simulink model "Comau_endeff_Comp"  (R2024b)
settings: Solver=FixedStepAuto  StartTime=0.0  StopTime=inf  FixedStep=Ts  RelTol=1e-3
model workspace (MATLAB code in the model file):
  | %% SMART_5NJ_110_3_0_DataFile
  | %============= RigidTransform =============%
  | 
  | %Initialize the RigidTransform structure array by filling in null values.
  | smiDataRobot.RigidTransform(16).translation = [0.0 0.0 0.0];
  | smiDataRobot.RigidTransform(16).angle = 0.0;
  | smiDataRobot.RigidTransform(16).axis = [0.0 0.0 0.0];
  | smiDataRobot.RigidTransform(16).ID = "";
  | 
  | %Translation Method - Cartesian
  | %Rotation Method - Arbitrary Axis
  | smiDataRobot.RigidTransform(1).translation = [0 331 0];  % mm
  | smiDataRobot.RigidTransform(1).angle = 0;  % rad
  | smiDataRobot.RigidTransform(1).axis = [0 0 0];
  | smiDataRobot.RigidTransform(1).ID = "AssemblyGround[SMART-5 NJ-110-3.0 (3D-STEP).STEP-1:SMART-5 NJ-110-3.0_p02.STEP-1]";
  | 
  | %Translation Method - Cartesian
  | %Rotation Method - Arbitrary Axis
  | smiDataRobot.RigidTransform(2).translation = [-450 2240 0];  % mm
  | smiDataRobot.RigidTransform(2).angle = 0;  % rad
  | smiDataRobot.RigidTransform(2).axis = [0 0 0];
  | smiDataRobot.RigidTransform(2).ID = "AssemblyGround[SMART-5 NJ-110-3.0 (3D-STEP).STEP-1:SMART-5 NJ-110-3.0_p05.STEP-1]";
  | 
  | %Translation Method - Cartesian
  | %Rotation Method - Arbitrary Axis
  | smiDataRobot.RigidTransform(3).translation = [-350 830 294.75];  % mm
  | smiDataRobot.RigidTransform(3).angle = 3.1415926535897931;  % rad
  | smiDataRobot.RigidTransform(3).axis = [1 0 0];
  | smiDataRobot.RigidTransform(3).ID = "AssemblyGround[SMART-5 NJ-110-3.0 (3D-STEP).STEP-1:SMART-5 NJ-110-3.0_CR82350080_SM.STEP-1]";
  | 
  | %Translation Method - Cartesian
  | %Rotation Method - Arbitrary Axis
  | smiDataRobot.RigidTransform(4).translation = [-1842.1799999999998 2240 9.9999999999999998e-13];  % mm
  | smiDataRobot.RigidTransform(4).angle = 0;  % rad
  | smiDataRobot.RigidTransform(4).axis = [0 0 0];
  | smiDataRobot.RigidTransform(4).ID = "AssemblyGround[SMART-5 NJ-110-3.0 (3D-STEP).STEP-1:SMART-5 NJ-110-3.0_p08.STEP-1]";
  | 
  | %Translation Method - Cartesian
  | %Rotation Method - Arbitrary Axis
  | smiDataRobot.RigidTransform(5).translation = [-1917.4300000000001 2240 -4.9999999999999997e-12];  % mm
  | smiDataRobot.RigidTransform(5).angle = 1.5707963267948977;  % rad
  | smiDataRobot.RigidTransform(5).axis = [-1.4999999999999981e-15 -1 -1.4999999999999981e-15];
  | smiDataRobot.RigidTransform(5).ID = "AssemblyGround[SMART-5 NJ-110-3.0 (3D-STEP).STEP-1:SMART-5 NJ-110-3.0_CR82350030_SM.STEP-1]";
  | 
  | %Translation Method - Cartesian
  | %Rotation Method - Arbitrary Axis
  | smiDataRobot.RigidTransform(6).translation = [0 0 0];  % mm
  | smiDataRobot.RigidTransform(6).angle = 0;  % rad
  | smiDataRobot.RigidTransform(6).axis = [0 0 0];
  | smiDataRobot.RigidTransform(6).ID = "AssemblyGround[SMART-5 NJ-110-3.0 (3D-STEP).STEP-1:SMART-5 NJ-110-3.0_p01.STEP-1]";
  | 
  | %Translation Method - Cartesian
  | %Rotation Method - Arbitrary Axis
  | smiDataRobot.RigidTransform(7).translation = [-240.25 2190 169.72568626429799];  % mm
  | smiDataRobot.RigidTransform(7).angle = 2.0943951023931966;  % rad
  | smiDataRobot.RigidTransform(7).axis = [0.57735026918962562 -0.57735026918962606 -0.57735026918962562];
  | smiDataRobot.RigidTransform(7).ID = "AssemblyGround[SMART-5 NJ-110-3.0 (3D-STEP).STEP-1:SMART-5 NJ-110-3.0_CR82350050_SM.STEP-1]";
  | 
  | %Translation Method - Cartesian
  | %Rotation Method - Arbitrary Axis
  | smiDataRobot.RigidTransform(8).translation = [-350 830 135.5];  % mm
  | smiDataRobot.RigidTransform(8).angle = 0;  % rad
  | smiDataRobot.RigidTransform(8).axis = [0 0 0];
  | smiDataRobot.RigidTransform(8).ID = "AssemblyGround[SMART-5 NJ-110-3.0 (3D-STEP).STEP-1:SMART-5 NJ-110-3.0_p03.STEP-1]";
  | 
  | %Translation Method - Cartesian
  | %Rotation Method - Arbitrary Axis
  | smiDataRobot.RigidTransform(9).translation = [-350 830 -350.25];  % mm
  | smiDataRobot.RigidTransform(9).angle = 3.1415926535897913;  % rad
  | smiDataRobot.RigidTransform(9).axis = [-0 -0 -1];
  | smiDataRobot.RigidTransform(9).ID = "AssemblyGround[SMART-5 NJ-110-3.0 (3D-STEP).STEP-1:SMART-5 NJ-110-3.0_CR82350070_SM.STEP-2]";
  | 
  | %Translation Method - Cartesian
  | %Rotation Method - Arbitrary Axis
  | smiDataRobot.RigidTransform(10).translation = [-31.217696610640999 802.11016232075008 -179.5];  % mm
  | smiDataRobot.RigidTransform(10).angle = 0;  % rad
  | smiDataRobot.RigidTransform(10).axis = [0 0 0];
  | smiDataRobot.RigidTransform(10).ID = "AssemblyGround[SMART-5 NJ-110-3.0 (3D-STEP).STEP-1:SMART-5 NJ-110-3.0_p06.STEP-1]";
  | 
  | %Translation Method - Cartesian
  | %Rotation Method - Arbitrary Axis
  | smiDataRobot.RigidTransform(11).translation = [-350 830 -194.5];  % mm
  | smiDataRobot.RigidTransform(11).angle = 0.087266462599717279;  % rad
  | smiDataRobot.RigidTransform(11).axis = [0 -1.1451882774215491e-14 -1];
  | smiDataRobot.RigidTransform(11).ID = "AssemblyGround[SMART-5 NJ-110-3.0 (3D-STEP).STEP-1:SMART-5 NJ-110-3.0_p04.STEP-1]";
  | 
  | %Translation Method - Cartesian
  | %Rotation Method - Arbitrary Axis
  | smiDataRobot.RigidTransform(12).translation = [-2007.179999999981 2240.0000000000132 -6.4999999999999995e-11];  % mm
  | smiDataRobot.RigidTransform(12).angle = 0;  % rad
  | smiDataRobot.RigidTransform(12).axis = [0 0 0];
  | smiDataRobot.RigidTransform(12).ID = "AssemblyGround[SMART-5 NJ-110-3.0 (3D-STEP).STEP-1:SMART-5 NJ-110-3.0_p10.STEP-1]";
  | 
  | %Translation Method - Cartesian
  | %Rotation Method - Arbitrary Axis
  | smiDataRobot.RigidTransform(13).translation = [156.75059808498401 472.5 90.5];  % mm
  | smiDataRobot.RigidTransform(13).angle = 2.7734925708571119;  % rad
  | smiDataRobot.RigidTransform(13).axis = [0.1861567878973851 0.69474659060686583 -0.69474659060686583];
  | smiDataRobot.RigidTransform(13).ID = "AssemblyGround[SMART-5 NJ-110-3.0 (3D-STEP).STEP-1:SMART-5 NJ-110-3.0_CR82350070_SM.STEP-1]";
  | 
  | %Translation Method - Cartesian
  | %Rotation Method - Arbitrary Axis
  | smiDataRobot.RigidTransform(14).translation = [-1967.1799999999998 2239.9999999999964 -2.5000000000000001e-11];  % mm
  | smiDataRobot.RigidTransform(14).angle = 1.5707963267948954;  % rad
  | smiDataRobot.RigidTransform(14).axis = [-4.5000000000000005e-15 1 3.5000000000000001e-15];
  | smiDataRobot.RigidTransform(14).ID = "AssemblyGround[SMART-5 NJ-110-3.0 (3D-STEP).STEP-1:SMART-5 NJ-110-3.0_p09.STEP-1]";
  | 
  | %Translation Method - Cartesian
  | %Rotation Method - Arbitrary Axis
  | smiDataRobot.RigidTransform(15).translation = [-495 2239.9999999999982 -2.5000000000000001e-11];  % mm
  | smiDataRobot.RigidTransform(15).angle = 2.0943951023932024;  % rad
  | smiDataRobot.RigidTransform(15).axis = [-0.57735026918962851 -0.57735026918962118 0.57735026918962751];
  | smiDataRobot.RigidTransform(15).ID = "AssemblyGround[SMART-5 NJ-110-3.0 (3D-STEP).STEP-1:SMART-5 NJ-110-3.0_p07.STEP-1]";
  | 
  | %Translation Method - Cartesian
  | %Rotation Method - Arbitrary Axis
  | smiDataRobot.RigidTransform(16).translation = [0 0 0];  % mm
  | smiDataRobot.RigidTransform(16).angle = 0;  % rad
  | smiDataRobot.RigidTransform(16).axis = [0 0 0];
  | smiDataRobot.RigidTransform(16).ID = "RootGround[SMART-5 NJ-110-3.0 (3D-STEP).STEP-1]";
  | 
  | 
  | %============= Solid =============%
  | %Center of Mass (CoM) %Moments of Inertia (MoI) %Product of Inertia (PoI)
  | 
  | %Initialize the Solid structure array by filling in null values.
  | smiDataRobot.Solid(14).mass = 0.0;
  | smiDataRobot.Solid(14).CoM = [0.0 0.0 0.0];
  | smiDataRobot.Solid(14).MoI = [0.0 0.0 0.0];
  | smiDataRobot.Solid(14).PoI = [0.0 0.0 0.0];
  | smiDataRobot.Solid(14).color = [0.0 0.0 0.0];
  | smiDataRobot.Solid(14).opacity = 0.0;
  | smiDataRobot.Solid(14).ID = "";
  | 
  | %Inertia Type - Custom
  | %Visual Properties - Simple
  | smiDataRobot.Solid(1).mass = 52.706031176315982;  % kg
  | smiDataRobot.Solid(1).CoM = [-242.66897813542667 296.14549865714821 12.560965025190244];  % mm
  | smiDataRobot.Solid(1).MoI = [4136639.3686790983 3647453.6565928138 4173251.5664203875];  % kg*mm^2
  | smiDataRobot.Solid(1).PoI = [21269.015167562859 -54887.133975236575 1321088.2058438642];  % kg*mm^2
  | smiDataRobot.Solid(1).color = [0.203 0.210 0.239];
  | smiDataRobot.Solid(1).opacity = 1;
  | smiDataRobot.Solid(1).ID = "SMART-5 NJ-110-3.0_p02.STEP*:*Default";
  | 
  | %Inertia Type - Custom
  | %Visual Properties - Simple
  | smiDataRobot.Solid(2).mass = 25.314195721014904;  % kg
  | smiDataRobot.Solid(2).CoM = [81.922886858874577 -33.833989402443976 14.448782406787638];  % mm
  | smiDataRobot.Solid(2).MoI = [783008.26269064494 548584.67016851983 525604.1322728931];  % kg*mm^2
  | smiDataRobot.Solid(2).PoI = [-112599.38170428496 21299.174138007162 72588.874515329284];  % kg*mm^2
  | smiDataRobot.Solid(2).color = [0.792156862745098 0.81960784313725488 0.93333333333333335];
  | smiDataRobot.Solid(2).opacity = 1;
  | smiDataRobot.Solid(2).ID = "SMART-5 NJ-110-3.0_p05.STEP*:*Default";
  | 
  | %Inertia Type - Custom
  | %Visual Properties - Simple
  | smiDataRobot.Solid(3).mass = 9.4493198216073964;  % kg
  | smiDataRobot.Solid(3).CoM = [0.00035605587580101627 0.59254727846081734 -131.34248514352112];  % mm
  | smiDataRobot.Solid(3).MoI = [96683.905101085853 96090.527287838268 47612.014811029614];  % kg*mm^2
  | smiDataRobot.Solid(3).PoI = [678.15178926669853 -1.9373731491872181 -0.37884372181229253];  % kg*mm^2
  | smiDataRobot.Solid(3).color = [0.792156862745098 0.81960784313725488 0.93333333333333335];
  | smiDataRobot.Solid(3).opacity = 1;
  | smiDataRobot.Solid(3).ID = "SMART-5 NJ-110-3.0_CR82350080_SM.STEP*:*Default";
  | 
  | %Inertia Type - Custom
  | %Visual Properties - Simple
  | smiDataRobot.Solid(4).mass = 27.907822986627043;  % kg
  | smiDataRobot.Solid(4).CoM = [176.91381036358237 3.8341896469272663 1.9754510358205102];  % mm
  | smiDataRobot.Solid(4).MoI = [482005.2410957645 820993.89522460627 552912.66986302414];  % kg*mm^2
  | smiDataRobot.Solid(4).PoI = [-5805.283149630598 -66627.605911827952 -6375.7492384737961];  % kg*mm^2
  | smiDataRobot.Solid(4).color = [0.792156862745098 0.81960784313725488 0.93333333333333335];
  | smiDataRobot.Solid(4).opacity = 1;
  | smiDataRobot.Solid(4).ID = "SMART-5 NJ-110-3.0_p08.STEP*:*Default";
  | 
  | %Inertia Type - Custom
  | %Visual Properties - Simple
  | smiDataRobot.Solid(5).mass = 1.8204370609575367;  % kg
  | smiDataRobot.Solid(5).CoM = [0.0011781120658499607 1.8532136422554566 -83.079832406507592];  % mm
  | smiDataRobot.Solid(5).MoI = [7475.3672830480818 7269.0527134527229 2858.8228291073215];  % kg*mm^2
  | smiDataRobot.Solid(5).PoI = [189.23833790092377 0.076539858692730889 -0.14274057644209939];  % kg*mm^2
  | smiDataRobot.Solid(5).color = [0.792156862745098 0.81960784313725488 0.93333333333333335];
  | smiDataRobot.Solid(5).opacity = 1;
  | smiDataRobot.Solid(5).ID = "SMART-5 NJ-110-3.0_CR82350030_SM.STEP*:*Default";
  | 
  | %Inertia Type - Custom
  | %Visual Properties - Simple
  | smiDataRobot.Solid(6).mass = 98.712536679746705;  % kg
  | smiDataRobot.Solid(6).CoM = [36.183943831325131 132.25114554111747 -0.030525648643372944];  % mm
  | smiDataRobot.Solid(6).MoI = [3268478.8711421788 6102276.4254572866 4269111.0143532446];  % kg*mm^2
  | smiDataRobot.Solid(6).PoI = [-35.583053939592197 631.47068636807955 -2524.4017230519235];  % kg*mm^2
  | smiDataRobot.Solid(6).color = [0.792156862745098 0.81960784313725488 0.93333333333333335];
  | smiDataRobot.Solid(6).opacity = 1;
  | smiDataRobot.Solid(6).ID = "SMART-5 NJ-110-3.0_p01.STEP*:*Default";
  | 
  | %Inertia Type - Custom
  | %Visual Properties - Simple
  | smiDataRobot.Solid(7).mass = 3.5666359355844257;  % kg
  | smiDataRobot.Solid(7).CoM = [1.2461000205248818 -0.0010192432622059655 -85.200466358919499];  % mm
  | smiDataRobot.Solid(7).MoI = [17145.157040564802 17509.336534066519 10295.619245635809];  % kg*mm^2
  | smiDataRobot.Solid(7).PoI = [-0.163954126982988 300.11359564551077 0.32104894325969818];  % kg*mm^2
  | smiDataRobot.Solid(7).color = [0.6392157 0.0 0.0];
  | smiDataRobot.Solid(7).opacity = 1;
  | smiDataRobot.Solid(7).ID = "SMART-5 NJ-110-3.0_CR82350050_SM.STEP*:*Default";
  | 
  | %Inertia Type - Custom
  | %Visual Properties - Simple
  | smiDataRobot.Solid(8).mass = 22.854890403146104;  % kg
  | smiDataRobot.Solid(8).CoM = [-23.928506665749911 523.99566525340538 -159.70044895169784];  % mm
  | smiDataRobot.Solid(8).MoI = [3177590.9155515293 341455.30737882649 3069690.399421786];  % kg*mm^2
  | smiDataRobot.Solid(8).PoI = [51188.540610659591 -6971.0396180961588 7197.3923801430437];  % kg*mm^2
  | smiDataRobot.Solid(8).color = [0.64 0.0 0.0];
  | smiDataRobot.Solid(8).opacity = 1;
  | smiDataRobot.Solid(8).ID = "SMART-5 NJ-110-3.0_p03.STEP*:*Default";
  | 
  | %Inertia Type - Custom
  | %Visual Properties - Simple
  | smiDataRobot.Solid(9).mass = 8.5814594224327365;  % kg
  | smiDataRobot.Solid(9).CoM = [0.00039190881468678792 0.65247306493897117 -117.33220651590989];  % mm
  | smiDataRobot.Solid(9).MoI = [76220.255867257161 75627.213475154422 43301.239657847611];  % kg*mm^2
  | smiDataRobot.Solid(9).PoI = [598.99194041261785 -1.5272912821901943 -0.37849880267797315];  % kg*mm^2
  | smiDataRobot.Solid(9).color = [0.792156862745098 0.81960784313725488 0.93333333333333335];
  | smiDataRobot.Solid(9).opacity = 1;
  | smiDataRobot.Solid(9).ID = "SMART-5 NJ-110-3.0_CR82350070_SM.STEP*:*Default";
  | 
  | %Inertia Type - Custom
  | %Visual Properties - Simple
  | smiDataRobot.Solid(10).mass = 7.5792666918117497;  % kg
  | smiDataRobot.Solid(10).CoM = [65.147048462687252 508.83792056545542 14.747257945702893];  % mm
  | smiDataRobot.Solid(10).MoI = [667373.64067244437 18083.172326137388 678945.36689657171];  % kg*mm^2
  | smiDataRobot.Solid(10).PoI = [-225.7042116055666 46.998810275833364 17500.803228922214];  % kg*mm^2
  | smiDataRobot.Solid(10).color = [0.792156862745098 0.81960784313725488 0.93333333333333335];
  | smiDataRobot.Solid(10).opacity = 1;
  | smiDataRobot.Solid(10).ID = "SMART-5 NJ-110-3.0_p06.STEP*:*Default";
  | 
  | %Inertia Type - Custom
  | %Visual Properties - Simple
  | smiDataRobot.Solid(11).mass = 4.3287759696132397;  % kg
  | smiDataRobot.Solid(11).CoM = [163.57070996069299 -9.8617817182830834 27.536485713357724];  % mm
  | smiDataRobot.Solid(11).MoI = [15456.864188549995 65374.86371961276 72810.661297813465];  % kg*mm^2
  | smiDataRobot.Solid(11).PoI = [-165.91415506329329 512.48565629209236 3817.7544015007338];  % kg*mm^2
  | smiDataRobot.Solid(11).color = [0.792156862745098 0.81960784313725488 0.93333333333333335];
  | smiDataRobot.Solid(11).opacity = 1;
  | smiDataRobot.Solid(11).ID = "SMART-5 NJ-110-3.0_p04.STEP*:*Default";
  | 
  | %Inertia Type - Custom
  | %Visual Properties - Simple
  | smiDataRobot.Solid(12).mass = 0.47985825240457192;  % kg
  | smiDataRobot.Solid(12).CoM = [-27.34791626851143 -1.6026209534547153 -5.1001180974803206e-05];  % mm
  | smiDataRobot.Solid(12).MoI = [1618.4776017805987 894.29456427734294 837.21364973354628];  % kg*mm^2
  | smiDataRobot.Solid(12).PoI = [-7.7780608542633322e-06 0.00054638186946613686 4.4070273941284572];  % kg*mm^2
  | smiDataRobot.Solid(12).color = [0.792156862745098 0.81960784313725488 0.93333333333333335];
  | smiDataRobot.Solid(12).opacity = 1;
  | smiDataRobot.Solid(12).ID = "SMART-5 NJ-110-3.0_p10.STEP*:*Default";
  | 
  | %Inertia Type - Custom
  | %Visual Properties - Simple
  | smiDataRobot.Solid(13).mass = 2.1916043056807371;  % kg
  | smiDataRobot.Solid(13).CoM = [-0.46659407311739648 -0.96652135243620041 26.711273550845025];  % mm
  | smiDataRobot.Solid(13).MoI = [11436.827713254688 13423.173203473376 8596.8063115297427];  % kg*mm^2
  | smiDataRobot.Solid(13).PoI = [153.22479160131755 -298.20565802941911 -10.064478096809076];  % kg*mm^2
  | smiDataRobot.Solid(13).color = [0.792156862745098 0.81960784313725488 0.93333333333333335];
  | smiDataRobot.Solid(13).opacity = 1;
  | smiDataRobot.Solid(13).ID = "SMART-5 NJ-110-3.0_p09.STEP*:*Default";
  | 
  | %Inertia Type - Custom
  | %Visual Properties - Simple
  | smiDataRobot.Solid(14).mass = 18.744700041112438;  % kg
  | smiDataRobot.Solid(14).CoM = [-0.005958152306662661 -0.089401100201608463 460.33855874646821];  % mm
  | smiDataRobot.Solid(14).MoI = [1632832.4693022415 1632553.6239231301 67074.935683703909];  % kg*mm^2
  | smiDataRobot.Solid(14).PoI = [-835.38260715793831 53.677126594132538 -8.4899136334609864];  % kg*mm^2
  | smiDataRobot.Solid(14).color = [0.792156862745098 0.81960784313725488 0.93333333333333335];
  | smiDataRobot.Solid(14).opacity = 1;
  | smiDataRobot.Solid(14).ID = "SMART-5 NJ-110-3.0_p07.STEP*:*Default";
values from neighbouring files (symbols this model uses):
  BList = Adjoint(M_B) * SList    [Comau_robot_3dof_parameters.m]
  M = [1 0 0 L1+L5+L6+L7 ... (first row only)    [Comau_robot_3dof_parameters.m]
  M_B = TransInv(M)    [Comau_robot_3dof_parameters.m]
  SList = [omega_mat; v_mat]    [Comau_robot_3dof_parameters.m]
  thetaList0 = [0 0 0 0 0]    [Comau_robot_3dof_parameters.m]
  tr_p_c = [-1.082024099747949, 1.536041691521612, -0.3]    [Comau_robot_3dof_parameters.m]
  tr_w_p = [-2.969661622702265, 1.976311036084776, 3.312845015592614]    [Comau_robot_3dof_parameters.m]
undefined symbols (not defined in the file or in its folder): L2, L3, L4, SF_x, SF_y, SF_z, smiDataRobot, X, Y, Z
libraries: sm_lib x96, nesl_utility x69, slrealtimeutilitieslib x2, slrealtimeiplib x2, simulink x1, aerolibanimutils x1
(part 1 of 5)
settings Model: Creator=jojoa  LastModifiedBy=Thoma

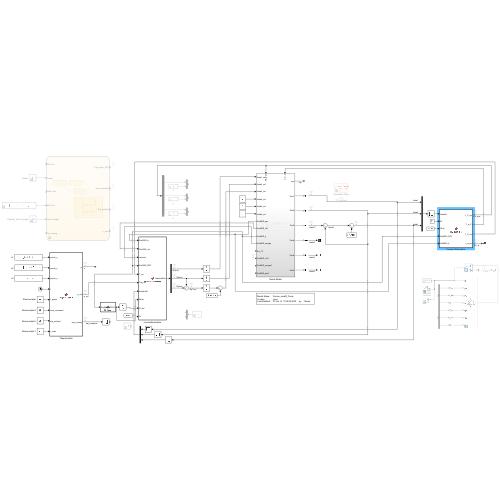
[thumbnail: Simulink's stored preview of the top-level diagram]
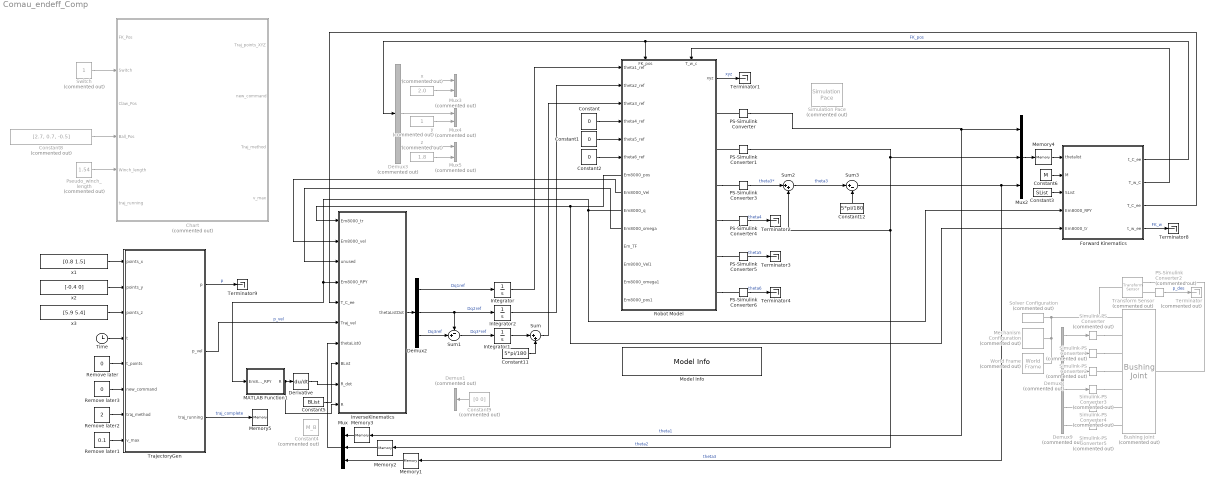
== system Comau_endeff_Comp ==
  Bushing Joint : sm_lib/Joints/Bushing Joint  Commented=on  JointMode=Normal  CompositeWrenchDir=FollowerOnBase  CompositeWrenchFrame=BaseFrame  SenseConstraintForce=off  SenseConstraintTorque=off  SenseTotalForce=off  SenseTotalTorque=off  PxPositionTargetSpecify=off  PxPositionTargetPriority=High  PxPositionTargetValue=0  PxPositionTargetValueUnits=m  PxVelocityTargetSpecify=off  PxVelocityTargetPriority=High  PxVelocityTargetValue=0  PxVelocityTargetValueUnits=m/s  PxEquilibriumPosition=0  PxEquilibriumPositionUnits=m  PxSpringStiffness=0  PxSpringStiffnessUnits=N/m  PxDampingCoefficient=0  PxDampingCoefficientUnits=N/(m/s)  PxLowerLimitSpecify=off  PxLowerLimitBound=-1  PxLowerLimitBoundUnits=m  PxLowerLimitStiffness=1e6  PxLowerLimitStiffnessUnits=N/m  PxLowerLimitDamping=1e3  PxLowerLimitDampingUnits=N/(m/s)  PxLowerLimitTransitionRegionWidth=1e-4  PxLowerLimitTransitionRegionWidthUnits=m  PxUpperLimitSpecify=off  PxUpperLimitBound=1  PxUpperLimitBoundUnits=m  PxUpperLimitStiffness=1e6  PxUpperLimitStiffnessUnits=N/m  PxUpperLimitDamping=1e3  PxUpperLimitDampingUnits=N/(m/s)  PxUpperLimitTransitionRegionWidth=1e-4  PxUpperLimitTransitionRegionWidthUnits=m  PxTorqueActuationMode=ComputedTorque  PxMotionActuationMode=InputMotion  PxSensePosition=off  PxSenseVelocity=off  PxSenseAcceleration=off  PxSenseTorqueForce=off  PxSenseLowerLimitTorqueForce=off  PxSenseUpperLimitTorqueForce=off  PyPositionTargetSpecify=off  PyPositionTargetPriority=High  PyPositionTargetValue=0  PyPositionTargetValueUnits=m  PyVelocityTargetSpecify=off  PyVelocityTargetPriority=High  PyVelocityTargetValue=0  PyVelocityTargetValueUnits=m/s  PyEquilibriumPosition=0  PyEquilibriumPositionUnits=m  PySpringStiffness=0  PySpringStiffnessUnits=N/m  PyDampingCoefficient=0  PyDampingCoefficientUnits=N/(m/s)  PyLowerLimitSpecify=off  PyLowerLimitBound=-1  PyLowerLimitBoundUnits=m  PyLowerLimitStiffness=1e6  PyLowerLimitStiffnessUnits=N/m  PyLowerLimitDamping=1e3  PyLowerLimitDampingUnits=N/(m/s)  PyLowerLimitTransitionRegionWidth=1e-4  PyLowerLimitTransitionRegionWidthUnits=m  PyUpperLimitSpecify=off  PyUpperLimitBound=1  PyUpperLimitBoundUnits=m  PyUpperLimitStiffness=1e6  PyUpperLimitStiffnessUnits=N/m  PyUpperLimitDamping=1e3  PyUpperLimitDampingUnits=N/(m/s)  PyUpperLimitTransitionRegionWidth=1e-4  PyUpperLimitTransitionRegionWidthUnits=m  PyTorqueActuationMode=ComputedTorque  PyMotionActuationMode=InputMotion  PySensePosition=off  PySenseVelocity=off  PySenseAcceleration=off  PySenseTorqueForce=off  PySenseLowerLimitTorqueForce=off  PySenseUpperLimitTorqueForce=off  PzPositionTargetSpecify=off  PzPositionTargetPriority=High  PzPositionTargetValue=0  PzPositionTargetValueUnits=m  PzVelocityTargetSpecify=off  PzVelocityTargetPriority=High  PzVelocityTargetValue=0  PzVelocityTargetValueUnits=m/s  PzEquilibriumPosition=0  PzEquilibriumPositionUnits=m  PzSpringStiffness=0  PzSpringStiffnessUnits=N/m  PzDampingCoefficient=0  PzDampingCoefficientUnits=N/(m/s)  PzLowerLimitSpecify=off  PzLowerLimitBound=-1  PzLowerLimitBoundUnits=m  PzLowerLimitStiffness=1e6  PzLowerLimitStiffnessUnits=N/m  PzLowerLimitDamping=1e3  PzLowerLimitDampingUnits=N/(m/s)  PzLowerLimitTransitionRegionWidth=1e-4  PzLowerLimitTransitionRegionWidthUnits=m  PzUpperLimitSpecify=off  PzUpperLimitBound=1  PzUpperLimitBoundUnits=m  PzUpperLimitStiffness=1e6  PzUpperLimitStiffnessUnits=N/m  PzUpperLimitDamping=1e3  PzUpperLimitDampingUnits=N/(m/s)  PzUpperLimitTransitionRegionWidth=1e-4  PzUpperLimitTransitionRegionWidthUnits=m  PzTorqueActuationMode=ComputedTorque  PzMotionActuationMode=InputMotion  PzSensePosition=off  PzSenseVelocity=off  PzSenseAcceleration=off  PzSenseTorqueForce=off  PzSenseLowerLimitTorqueForce=off  PzSenseUpperLimitTorqueForce=off  RxPositionTargetSpecify=off  RxPositionTargetPriority=High  RxPositionTargetValue=0  RxPositionTargetValueUnits=deg  RxVelocityTargetSpecify=off  RxVelocityTargetPriority=High  RxVelocityTargetValue=0  RxVelocityTargetValueUnits=deg/s  RxEquilibriumPosition=0  RxEquilibriumPositionUnits=deg  RxSpringStiffness=0  RxSpringStiffnessUnits=N*m/deg  RxDampingCoefficient=0  RxDampingCoefficientUnits=N*m/(deg/s)  RxLowerLimitSpecify=off  RxLowerLimitBound=-90  RxLowerLimitBoundUnits=deg  RxLowerLimitStiffness=1e4  RxLowerLimitStiffnessUnits=N*m/deg  RxLowerLimitDamping=10  RxLowerLimitDampingUnits=N*m/(deg/s)  RxLowerLimitTransitionRegionWidth=0.1  RxLowerLimitTransitionRegionWidthUnits=deg  RxUpperLimitSpecify=off  RxUpperLimitBound=90  RxUpperLimitBoundUnits=deg  RxUpperLimitStiffness=1e4  RxUpperLimitStiffnessUnits=N*m/deg  RxUpperLimitDamping=10  RxUpperLimitDampingUnits=N*m/(deg/s)  RxUpperLimitTransitionRegionWidth=0.1  RxUpperLimitTransitionRegionWidthUnits=deg  RxTorqueActuationMode=ComputedTorque  RxMotionActuationMode=InputMotion  RxSensePosition=off  RxSenseVelocity=off  RxSenseAcceleration=off  RxSenseTorqueForce=off  RxSenseLowerLimitTorqueForce=off  RxSenseUpperLimitTorqueForce=off  RyPositionTargetSpecify=off  RyPositionTargetPriority=High  RyPositionTargetValue=0  RyPositionTargetValueUnits=deg  RyVelocityTargetSpecify=off  RyVelocityTargetPriority=High  RyVelocityTargetValue=0  RyVelocityTargetValueUnits=deg/s  RyEquilibriumPosition=0  RyEquilibriumPositionUnits=deg  RySpringStiffness=0  RySpringStiffnessUnits=N*m/deg  RyDampingCoefficient=0  RyDampingCoefficientUnits=N*m/(deg/s)  RyLowerLimitSpecify=off  RyLowerLimitBound=-90  RyLowerLimitBoundUnits=deg  RyLowerLimitStiffness=1e4  RyLowerLimitStiffnessUnits=N*m/deg  RyLowerLimitDamping=10  RyLowerLimitDampingUnits=N*m/(deg/s)  RyLowerLimitTransitionRegionWidth=0.1  RyLowerLimitTransitionRegionWidthUnits=deg  RyUpperLimitSpecify=off  RyUpperLimitBound=90  RyUpperLimitBoundUnits=deg  RyUpperLimitStiffness=1e4  RyUpperLimitStiffnessUnits=N*m/deg  RyUpperLimitDamping=10  RyUpperLimitDampingUnits=N*m/(deg/s)  RyUpperLimitTransitionRegionWidth=0.1  RyUpperLimitTransitionRegionWidthUnits=deg  RyTorqueActuationMode=ComputedTorque  RyMotionActuationMode=InputMotion  RySensePosition=off  RySenseVelocity=off  RySenseAcceleration=off  RySenseTorqueForce=off  RySenseLowerLimitTorqueForce=off  RySenseUpperLimitTorqueForce=off  RzPositionTargetSpecify=off  RzPositionTargetPriority=High  RzPositionTargetValue=0  RzPositionTargetValueUnits=deg  RzVelocityTargetSpecify=off  RzVelocityTargetPriority=High  RzVelocityTargetValue=0  RzVelocityTargetValueUnits=deg/s  RzEquilibriumPosition=0  RzEquilibriumPositionUnits=deg  RzSpringStiffness=0  RzSpringStiffnessUnits=N*m/deg  RzDampingCoefficient=0  RzDampingCoefficientUnits=N*m/(deg/s)  RzLowerLimitSpecify=off  RzLowerLimitBound=-90  RzLowerLimitBoundUnits=deg  RzLowerLimitStiffness=1e4  RzLowerLimitStiffnessUnits=N*m/deg  RzLowerLimitDamping=10  RzLowerLimitDampingUnits=N*m/(deg/s)  RzLowerLimitTransitionRegionWidth=0.1  RzLowerLimitTransitionRegionWidthUnits=deg  RzUpperLimitSpecify=off  RzUpperLimitBound=90  RzUpperLimitBoundUnits=deg  RzUpperLimitStiffness=1e4  RzUpperLimitStiffnessUnits=N*m/deg  RzUpperLimitDamping=10  RzUpperLimitDampingUnits=N*m/(deg/s)  RzUpperLimitTransitionRegionWidth=0.1  RzUpperLimitTransitionRegionWidthUnits=deg  RzTorqueActuationMode=ComputedTorque  RzMotionActuationMode=InputMotion  RzSensePosition=off  RzSenseVelocity=off  RzSenseAcceleration=off  RzSenseTorqueForce=off  RzSenseLowerLimitTorqueForce=off  RzSenseUpperLimitTorqueForce=off
  Chart : Stateflow chart  Commented=on  TreatAsAtomicUnit=on
      settings: PortSchema="{\"entries\":[{\"content\":{\"sides\":[{\"content\":{\"connectorIds\":[\"In2\",\"In1\",\"In3\",\"In4\",\"In5\",\"In6\"]},\"type\":\"ConnectorPlacement.EquallySpacedRectSide\",\"uuid\":\"172fb156-0aeb-45d6-ae82-af15bd6c897e\"},{\"content\":{\"connectorIds\":[\"Out1\",\"Out2\",\"Out3\",\"Out4\"],\"side\":\"RIGHT\"},\"type\":\"ConnectorPlacement.EquallySpacedRectSide\",\"uuid\":\"236a4085-9b1e-46f1-9589-a1369625993a\"},{\"content\":{\"side\":\"TOP\"},\"type\":\"ConnectorPlacement.EquallySpacedRectSide\",\"uuid\":\"81d2e992-6e31-4ebe-a88a-0042095fc779\"}]},\"type\":\"ConnectorPlacement.EquallySpacedConnector\",\"uuid\":\"b030cd03-88b5-40ca-9a91-4cb72ee04091\"}],\"packageUris\":[\"http://schema.mathworks.com/mf0/Connector/R2020b\"],\"version\":\"1.0\"}"
  Constant : Constant  Value=0
  Constant1 : Constant  Value=0
  Constant11 : Constant  Value=5*pi/180
  Constant12 : Constant  Value=5*pi/180
  Constant2 : Constant  Value=0
  Constant3 : Constant  Value=SList
  Constant4 : Constant  Commented=on  Value=M_B
  Constant5 : Constant  Value=BList
  Constant6 : Constant  Value=M
  Constant8 : Constant  Commented=on  Value=[2.7, 0.7, -0.5]
  Constant9 : Constant  Commented=on  Value=[0 0]
  Demux1 : Demux  Commented=on  Outputs=2
  Demux2 : Demux  Outputs=3
  Demux3 : Demux  Commented=on  Outputs=3
  Demux8 : Demux  Commented=on  Outputs=3
  Demux9 : Demux  Commented=on  Outputs=3
  Derivative : Derivative
  Forward Kinematics : MATLAB Function  TreatAsAtomicUnit=on
  Integrator : Integrator
  Integrator1 : Integrator
  Integrator2 : Integrator
  MATLAB Function1 : MATLAB Function  TreatAsAtomicUnit=on
  Mechanism Configuration : sm_lib/Utilities/Mechanism Configuration  Commented=on  UniformGravity=Constant  GravityVector=[0 0 -9.80665]  GravityVectorUnits=m/s^2  LinearizationDelta=0.001  JointModeTransitionNonlinearIterations=2
  Memory1 : Memory  InitialCondition=thetaList0(3)
  Memory2 : Memory  InitialCondition=thetaList0(2)
  Memory3 : Memory  InitialCondition=thetaList0(1)
  Memory4 : Memory
  Memory5 : Memory
  Model Info : simulink/Model-Wide Utilities/Model Info  Frame=on  DisplayStringWithTags=|  HorizontalTextAlignment=Left  LeftAlignmentValue=0.02
      | Model Name:     %<ModelName>
      | Creator:              %<Creator>
      | Last Modified:    %<LastModificationDate>     by    %<LastModifiedBy>
  Mux : Mux  Inputs=3
  Mux2 : Mux  Inputs=3
  Mux3 : Mux  Commented=on  Inputs=2
  Mux4 : Mux  Commented=on  Inputs=2
  Mux5 : Mux  Commented=on  Inputs=2
  PS-Simulink Converter{,1,3..6} (6 alike) : nesl_utility/PS-Simulink Converter  PhysicalDomain=network_engine_domain  SubClassName=ps_output  LeftPortType=input  RightPortType=output  PseudoPeriodic=off  Frequencies=[]  VectorFormat=inherit  Unit=inherit  AffineConversion=off
  PS-Simulink Converter2 : nesl_utility/PS-Simulink Converter  Commented=on  PhysicalDomain=network_engine_domain  SubClassName=ps_output  LeftPortType=input  RightPortType=output  PseudoPeriodic=off  Frequencies=[]  VectorFormat=inherit  Unit=inherit  AffineConversion=off
  Pseudo_winch_length : Constant  Commented=on  Value=1.54
  Remove later : Constant  Value=0
  Remove later1 : Constant  Value=0.1
  Remove later2 : Constant  Value=2
  Remove later3 : Constant  Value=0
  Robot Model : Subsystem
      settings: PortSchema="{\"entries\":[{\"content\":{\"sides\":[{\"content\":{\"connectorIds\":[\"In1\",\"In2\",\"In3\",\"In4\",\"In5\",\"In6\",\"Out2\",\"Out3\",\"Out4\",\"Out5\",\"Out6\",\"Out7\",\"Out8\",\"Out9\"]},\"type\":\"ConnectorPlacement.EquallySpacedRectSide\",\"uuid\":\"6aa2e516-c804-4755-b4dc-c78d50aa59d9\"},{\"content\":{\"connectorIds\":[\"Out1\",\"RConn1\",\"RConn2\",\"RConn3\",\"RConn4\",\"RConn5\",\"RConn6\"],\"side\":\"RIGHT\"},\"type\":\"ConnectorPlacement.EquallySpacedRectSide\",\"uuid\":\"639c1142-9616-4d5f-b210-c20b0bbda392\"},{\"content\":{\"connectorIds\":[\"In7\",\"In8\"],\"side\":\"TOP\"},\"type\":\"ConnectorPlacement.EquallySpacedRectSide\",\"uuid\":\"5b61a740-c71f-4d58-86f2-86cfe83aa5ec\"}]},\"type\":\"ConnectorPlacement.EquallySpacedConnector\",\"uuid\":\"c7a9e42c-08d7-4193-b201-c243b42c995e\"}],\"packageUris\":[\"http://schema.mathworks.com/mf0/Connector/R2020b\"],\"version\":\"1.0\"}"
  Simulation Pace : aerolibanimutils/Simulation Pace  Commented=on  SimulationPace=1  SleepMode=Auto  OutputPaceError=off  SampleTime=0.001
  Simulink-PS Converter{,1..5} (6 alike) : nesl_utility/Simulink-PS Converter  Commented=on  PhysicalDomain=network_engine_domain  SubClassName=ps_input  LeftPortType=input  RightPortType=output  PseudoPeriodic=off  Frequencies=[]  NoiseDistribution=none  NoiseParameters=[]  Unit=1  AffineConversion=off  FilteringAndDerivatives=filter  SimscapeFilterOrder=2  InputFilterTimeConstant=0.001  UdotUserProvided=0
  Solver Configuration : nesl_utility/Solver Configuration  Commented=on  PhysicalDomain=network_engine_domain  SubClassName=solver  LeftPortType=input  RightPortType=generic  Tones=[]  Harmonics=[]  SimulateNoise=off  Profile=off  UseLocalSampling=off  EnableSwitchedLinearOptims=on  FrequencyDomain=off  UseCCode=off  RelTol=0.001  AbsTol=0.001  MinStep=1e-09  ToWorkspace=off  RevertToSquareIcSolve=off  NumHomotopyIterations=100  PhasorMode=off  PhasorModeNumHarmonics=1  ConsistencySolver=NEWTON_XTOL_AFTER_FTOL  IndexReductionMethod=DerivativeReplacement  DoDC=off  ResidualTolerance=1e-09  ConsistencyTolSource=GLOBAL  ConsistencyAbsTol=0.001  ConsistencyRelTol=0.001  ConsistencyTolFactor=0.001  UseLocalSolver=off  LocalSolverChoice=NE_BACKWARD_EULER_ADVANCER  ResolveIndetEquations=on  FunctionEvalNumThread=1  LocalSolverSampleTime=0.001  DoFixedCost=off  MaxNonlinIter=3  MaxModeIter=2  ComputeImpulses=off  ImpulseIterations=2  LinearAlgebra=auto  LinearAlgebraNumThread=0  EquationFormulation=NE_TIME_EF  DelaysMemoryBudget=1024  AutomaticFiltering=on  FilteringTimeConstant=0.001  PartitionStorageMethod=AS_NEEDED  PartitionMemoryBudget=1024  PartitionMethod=ROBUST  MultibodyUseLocalSolver=off  MultibodyLocalSolverChoice=ODE1  MultibodyLocalSolverSampleTime=0.001
  Sum : Sum  Inputs=|++
  Sum1 : Sum  Inputs=-+|
  Sum2 : Sum  Inputs=|++
  Sum3 : Sum  Inputs=|+-
  Switch : Constant  Commented=on
  Terminator : Terminator  Commented=on
  Terminator{1..4,8..9} (6 alike) : Terminator
  Time : Clock
  TrajectoryGen : MATLAB Function  TreatAsAtomicUnit=on
  Transform Sensor : sm_lib/Frames and Transforms/Transform Sensor  Commented=on  MeasurementFrame=World  RotationSequence=XYX  SenseAngle=off  SenseAxis=off  SenseQ=off  SenseR=off  SenseRotationSequence=off  SenseOmegaX=off  SenseOmegaY=off  SenseOmegaZ=off  SenseOmega=off  SenseQDot=off  SenseRDot=off  SenseRotationSequenceDot=off  SenseAlphaX=off  SenseAlphaY=off  SenseAlphaZ=off  SenseAlpha=off  SenseQDDot=off  SenseRDDot=off  SenseX=off  SenseY=off  SenseZ=off  SenseXYZ=on  SenseRad=off  SenseAzim=off  SenseDist=off  SenseInc=off  SenseXDot=off  SenseYDot=off  SenseZDot=off  SenseXYZDot=off  SenseRadDot=off  SenseAzimDot=off  SenseDistDot=off  SenseIncDot=off  SenseXDDot=off  SenseYDDot=off  SenseZDDot=off  SenseXYZDDot=off  SenseRadDDot=off  SenseAzimDDot=off  SenseDistDDot=off  SenseIncDDot=off
  World Frame : sm_lib/Frames and Transforms/World Frame  Commented=on
  inverseKinematics : MATLAB Function  TreatAsAtomicUnit=on
  x : Constant  Commented=on  Value=2.0
  x1 : Constant  Value=[0.8 1.5]
  x2 : Constant  Value=[-0.4 0]
  x3 : Constant  Value=[5.9 5.4]
  y : Constant  Commented=on
  z : Constant  Commented=on  Value=1.8
  wires:
  PS-Simulink Converter/1 -> Memory3/1, Mux2/1  "theta1"
  Robot Model/1(xyz) -> Terminator1/1  "xyz"
  Mux/1 -> inverseKinematics/7(thetaList0)
  Memory3/1 -> Mux/1
  Constant5/1 -> inverseKinematics/8(BList)
  Memory2/1 -> Mux/2
  Demux2/1 -> Integrator/1  "Dq1ref"
  Constant/1 -> Robot Model/4(theta4_ref)
  Constant1/1 -> Robot Model/5(theta5_ref)
  Constant2/1 -> Robot Model/6(theta6_ref)
  Demux2/2 -> Sum1/1, Integrator2/1  "Dq2ref"
  Mux2/1 -> Memory4/1
  Constant6/1 -> Forward Kinematics/2(M)
  Constant3/1 -> Forward Kinematics/3(SList)
  PS-Simulink Converter4/1 -> Terminator2/1  "theta4"
  PS-Simulink Converter5/1 -> Terminator3/1  "theta5"
  PS-Simulink Converter6/1 -> Terminator4/1  "theta6"
  Time/1 -> TrajectoryGen/4(t)
  PS-Simulink Converter1/1 -> Memory2/1, Sum2/2, Mux2/2  "theta2"
  Memory1/1 -> Mux/3
  PS-Simulink Converter3/1 -> Sum2/1  "theta3*"
  Sum1/1 -> Integrator1/1  "Dq3*ref"
  Demux2/3 -> Sum1/2  "Dq3ref"
  Constant11/1 -> Sum/2
  Sum2/1 -> Sum3/1  "theta3"
  Constant12/1 -> Sum3/2
  Sum3/1 -> Memory1/1, Mux2/3  "theta3"
  Forward Kinematics/1(t_C_ee) -> Robot Model/7(FK_pos), Demux3/1  "FK_pos"
  Memory4/1 -> Forward Kinematics/1(thetalist)
  x/1 -> Mux3/2
  Demux3/1 -> Mux3/1
  Demux3/2 -> Mux4/1
  y/1 -> Mux4/2
  Demux3/3 -> Mux5/1
  z/1 -> Mux5/2
  Remove later/1 -> TrajectoryGen/5(t_points)
  Switch/1 -> Chart/1(Switch)
  Sum/1 -> Robot Model/3(theta3_ref)
  TrajectoryGen/3(traj_running) -> Memory5/1  "traj_complete"
  Pseudo_winch_length/1 -> Chart/5(Winch_length)
  Constant8/1 -> Chart/4(Ball_Pos)
  Remove later1/1 -> TrajectoryGen/8(v_max)
  Remove later2/1 -> TrajectoryGen/7(traj_method)
  Remove later3/1 -> TrajectoryGen/6(new_command)
  x1/1 -> TrajectoryGen/1(points_x)
  x2/1 -> TrajectoryGen/2(points_y)
  x3/1 -> TrajectoryGen/3(points_z)
  Demux8/1 -> Simulink-PS Converter/1
  Demux8/2 -> Simulink-PS Converter1/1
  Demux8/3 -> Simulink-PS Converter2/1
  Demux9/1 -> Simulink-PS Converter3/1
  Demux9/2 -> Simulink-PS Converter4/1
  Demux9/3 -> Simulink-PS Converter5/1
  PS-Simulink Converter2/1 -> Terminator/1  "p_des"
  Integrator1/1 -> Sum/1
  Integrator/1 -> Robot Model/1(theta1_ref)
  Integrator2/1 -> Robot Model/2(theta2_ref)
  Robot Model/2(Em8000_pos) -> Forward Kinematics/5(Em8000_tr), inverseKinematics/1(Em8000_tr)
  Robot Model/3(Em8000_Vel) -> inverseKinematics/2(Em8000_vel)
  Robot Model/5(Em8000_omega) -> inverseKinematics/3(unused)
  Robot Model/4(Em8000_q) -> MATLAB Function1/1(Em8000_RPY), inverseKinematics/4(Em8000_RPY), Forward Kinematics/4(Em8000_RPY)
  Forward Kinematics/3(T_C_ee) -> inverseKinematics/5(T_C_ee)
  inverseKinematics/1(thetaListDot) -> Demux2/1
  TrajectoryGen/2(p_vel) -> inverseKinematics/6(Traj_vel)  "p_vel"
  Constant9/1 -> Demux1/1
  Forward Kinematics/4(t_w_ee) -> Terminator8/1  "FK_w"
  TrajectoryGen/1(p) -> Terminator9/1  "p"
  MATLAB Function1/1(R) -> inverseKinematics/10(R), Derivative/1
  Derivative/1 -> inverseKinematics/9(R_dot)
  Forward Kinematics/2(T_w_C) -> Robot Model/8(T_w_c)
  connections:
  Robot Model/RConn4 -- PS-Simulink Converter4/LConn1
  PS-Simulink Converter/LConn1 -- Robot Model/RConn1
  Robot Model/RConn5 -- PS-Simulink Converter5/LConn1
  Robot Model/RConn3 -- PS-Simulink Converter3/LConn1
  PS-Simulink Converter1/LConn1 -- Robot Model/RConn2
  Robot Model/RConn6 -- PS-Simulink Converter6/LConn1
  World Frame/RConn1 -- Transform Sensor/LConn1 -- Bushing Joint/LConn1 -- Solver Configuration/RConn1 -- Mechanism Configuration/RConn1
  Simulink-PS Converter3/RConn1 -- Bushing Joint/LConn5
  Simulink-PS Converter4/RConn1 -- Bushing Joint/LConn6
  Simulink-PS Converter5/RConn1 -- Bushing Joint/LConn7
  Simulink-PS Converter1/RConn1 -- Bushing Joint/LConn3
  Simulink-PS Converter2/RConn1 -- Bushing Joint/LConn4
  Simulink-PS Converter/RConn1 -- Bushing Joint/LConn2
  Transform Sensor/RConn1 -- Bushing Joint/RConn1
  PS-Simulink Converter2/LConn1 -- Transform Sensor/RConn2
